simulink model "test"  (Simulink 4.00)
settings: Solver=FixedStepDiscrete  SolverMode=SingleTasking  StartTime=0.0  StopTime=999999  RelTol=1e-3  AbsTol=1e-6
libraries: dspsnks3 x3, dspsigattribs x2, dspsrcs3 x2, dspindex x1, dspadpt3 x1, dspddes3 x1, dspbuff3 x1
Description:
  | LMS adaptive noise cancellation
settings Model: CovMetricSettings=d  Creator=don  LastModifiedBy=admin  SaveTime=off  SaveOutput=off  IntegerOverflowMsg=none  ExtModeTrigMode=oneshot  ExtModeArmWhenConnect=off  BlockReductionOpt=off

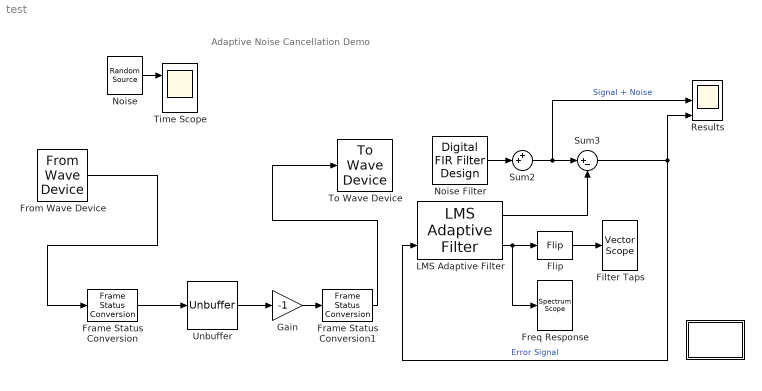
== system test ==
  note: Adaptive Noise Cancellation Demo
  " " : Subsystem
      settings: RTWFcnNameOpts=Auto  RTWFileNameOpts=Auto
      mask Display: disp('Info')
  Filter Taps : dspsnks3/Vector Scope  ScopeProperties=on  Domain=User-defined  HorizSpan=1  DisplayProperties=off  AxisGrid=on  Memory=off  FrameNumber=on  AxisLegend=off  AxisZoom=on  OpenScopeAtSimStart=on  OpenScopeImmediately=off  FigPos=[66 155 329 270]  AxisProperties=off  XUnits=Hertz  XRange=[0...Fs/2]  InheritXIncr=on  XIncr=1  XLabel=Samples  YUnits=dB  YLabel=Filter Coefficients  LineProperties=off  LineDisables=on  LineStyles=:  LineMarkers=.  LineColors=[0 0 1]
      settings: YMin=-0.2  YMax=0.6
  Flip : dspindex/Flip  dim=Columns
  Frame Status Conversion : dspsigattribs/Frame Status Conversion  growRefPort=off  outframe=Sample-based
  Frame Status Conversion1 : dspsigattribs/Frame Status Conversion  growRefPort=off  outframe=Frame-based
  Freq Response : dspsnks3/Spectrum Scope  ScopeProperties=on  Domain=Frequency  HorizSpan=1  UseBuffer=off  BufferSize=128  Overlap=64  inpFftLenInherit=on  FFTlength=256  numAvg=2  DisplayProperties=off  AxisGrid=on  Memory=off  FrameNumber=off  AxisLegend=off  AxisZoom=on  OpenScopeAtSimStart=on  OpenScopeImmediately=off  FigPos=[404 155 378 270]  AxisProperties=off  XUnits=Hertz  XRange=[0...Fs/2]  InheritXIncr=on  XIncr=1  XLabel=Samples  YUnits=dB  YLabel=Magnitude, dB  LineProperties=off  LineDisables=on  LineStyles=-  LineColors=[0 0 1]
      settings: YMin=-60  YMax=0
  From Wave Device : dspsrcs3/From Wave Device  SampleRate=8000  UserRate=16000  SampleWidth=8  Stereo=off  SamplesPerFrame=64  QueueDuration=2  useDefaultDevice=on  userDeviceID=1
  Gain : Gain  Gain=-1  Multiplication=Element-wise(K.*u)  SaturateOnIntegerOverflow=on
  LMS Adaptive Filter : dspadpt3/LMS Adaptive Filter  n=32  mu=0.5  ic=0.0  leakage=1.0  normalized=on  Adapt=off
  Noise : dspsrcs3/Random Source  SrcType=Gaussian  Min=0  Max=1  Mean=0  Var=1  RepMode=Specify seed  Seed=[23341]  Inherit=off  SampMode=Discrete  SampTime=1  SampFrame=1  OutComplex=Real
  Noise Filter : dspddes3/Digital FIR Filter Design  filttype=Lowpass  N=31  Wlo=0.5  Whi=0.6  W0=[.2 .5 .8]  g0=1  W1=[0 .2 .3 .6 .8 1]  gains=[1 .5 0 0 1 .5]  wintype=Hamming  Rs=10  Kbeta=5
  Results : Scope  NumInputPorts=3
      settings: TimeRange=399999.6  YMin=-2~-0.002166666666666664~-0.001  YMax=2~-0.001833333333333326~0.001  SaveToWorkspace=off  SaveName=ScopeData  DataFormat=Array  MaxDataPoints=5000
  Sum2 : Sum  Inputs=++|  SaturateOnIntegerOverflow=on
  Sum3 : Sum  Inputs=|+-  SaturateOnIntegerOverflow=on
  Time Scope : Scope  NumInputPorts=2
      settings: TimeRange=auto  YMin=0.338693~-0.035  YMax=0.374345~0.02  SaveToWorkspace=off  DataFormat=Structure  MaxDataPoints=5000
  To Wave Device : dspsnks3/To Wave Device  bufDuration=2  initDelay=0.1  useDefaultDevice=on  userDeviceID=1
  Unbuffer : dspbuff3/Unbuffer  ic=1
  wires:
  ? -> Sum2/1, Results/1  "Input Signal"
  Noise Filter/1 -> Sum2/2
  Sum2/1 -> Results/2, Sum3/1  "Signal + Noise"
  LMS Adaptive Filter/1 -> Sum3/2
  LMS Adaptive Filter/2 -> Freq Response/1, Flip/1
  Sum3/1 -> Results/3, LMS Adaptive Filter/2  "Error Signal"
  Flip/1 -> Filter Taps/1
  Noise/1 -> Time Scope/1
  From Wave Device/1 -> Frame Status Conversion/1
  Frame Status Conversion/1 -> Unbuffer/1
  Unbuffer/1 -> Gain/1
  Gain/1 -> Frame Status Conversion1/1
  Frame Status Conversion1/1 -> To Wave Device/1

== system test/  ==
  note: Adaptive Noise Cancellation using the Least
      | Mean Square Algorithm
      |
      | The LMS adaptive filter uses the reference signal (on
      | the "In" port) and the error signal (on the "Err" port) to automatically
      |  match the filter response in the block labeled "Noise filter".
      |  As it converges to the correct filter, the filtered noise should
      |  be completely subtracted from the "Signal + Noise" signal and
      | the "Error Signal" should contain only the original signal.
      |
      | For details, see "Adaptive Filter Theory", 3rd Ed. by
      | S. Haykin, Prentice-Hall 1996.
